simulink model "ball"  (R2017a)
settings: Solver=ode45  StartTime=0.0  StopTime=10.0  RelTol=1e-3
values from neighbouring files (symbols this model uses):
  g = -9.81    [stepinfo.m]
undefined symbols (not defined in the file or in its folder): d, J, L, m, R
settings Model: Creator=sansh  LastModifiedBy=sansh

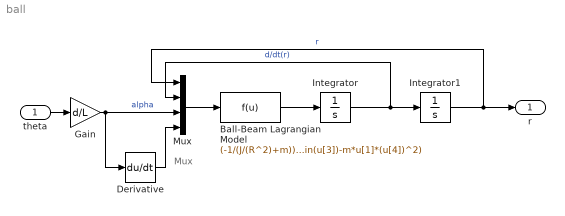
== system ball ==
  note: Mux
  theta : Inport
  Ball-Beam Lagrangian Model : Fcn  Expr=(-1/(J/(R^2)+m))*(m*g*sin(u[3])-m*u[1]*(u[4])^2)
  Derivative : Derivative
  Gain : Gain  Gain=d/L
  Integrator : Integrator
  Integrator1 : Integrator
  Mux : Mux
  r : Outport
  wires:
  Integrator/1 -> Mux/2, Integrator1/1  "d/dt(r)"
  Integrator1/1 -> Mux/1, r/1  "r"
  Ball-Beam Lagrangian Model/1 -> Integrator/1
  Mux/1 -> Ball-Beam Lagrangian Model/1
  theta/1 -> Gain/1
  Gain/1 -> Derivative/1, Mux/3  "alpha"
  Derivative/1 -> Mux/4
